simulink model "missile71"  (Simulink 6.3)
settings: Solver=ode4  StartTime=0.0  StopTime=10.0  FixedStep=0.0001  RelTol=1e-3
values from neighbouring files (symbols this model uses):
  K2 = lfr(D11,D12,D21,D22,blk)    [ex_2_1.m]
  Ma = 2 + jj*(2/5)    [ex_6_5_loop.m]
undefined symbols (not defined in the file or in its folder): K1, K3, m0, m1, m2, m3, z0, z1, z2, z3
settings Model: Creator=magni  LastModifiedBy=magni  ExtModeTrigMode=oneshot  ExtModeArmWhenConnect=off  ExtModeAutoUpdateStatusClock=off  StrictBusMsg=None
settings DataIOCC: LimitDataPoints=off
settings OptimizationCC: BlockReduction=off  BooleanDataType=off
settings DebuggingCC: SolverPrmCheckMsg=none
settings HardwareCC: TargetUnknown=on

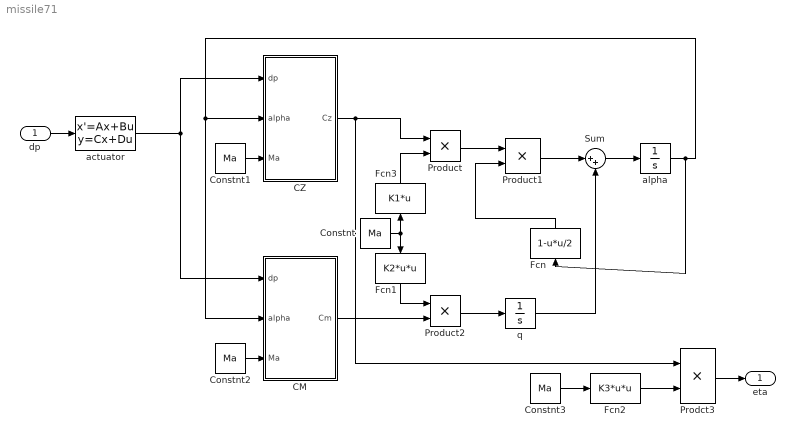
== system missile71 ==
  dp : Inport
  CM : Subsystem
  CZ : Subsystem
  Constnt{,1..3} (4 alike) : Constant  Value=Ma
  Fcn : Fcn  Orientation=up  Expr=1-u*u/2
  Fcn1 : Fcn  Orientation=down  Expr=K2*u*u
  Fcn2 : Fcn  Expr=K3*u*u
  Fcn3 : Fcn  Orientation=up  Expr=K1*u
  Prodct3 : Product  SaturateOnIntegerOverflow=on  RndMeth=Zero  InputSameDT=on
  Product : Product  SaturateOnIntegerOverflow=on  RndMeth=Zero  InputSameDT=on
  Product1 : Product  SaturateOnIntegerOverflow=on  RndMeth=Zero  InputSameDT=on
  Product2 : Product  SaturateOnIntegerOverflow=on  RndMeth=Zero  InputSameDT=on
  Sum : Sum  Inputs=|++  SaturateOnIntegerOverflow=on  InputSameDT=on
  actuator : StateSpace  A=[-210 -175.8;128 0]  B=[16;0]  C=[0 10.98]  D=0  X0=[0;0]
  alpha : Integrator
  q : Integrator
  eta : Outport
  wires:
  q/1 -> Sum/2
  Fcn3/1 -> Product/2
  Fcn/1 -> Product1/2
  Product/1 -> Product1/1
  Product1/1 -> Sum/1
  Sum/1 -> alpha/1
  Fcn1/1 -> Product2/1
  CM/1(Cm) -> Product2/2
  Product2/1 -> q/1
  CZ/1(Cz) -> Product/1, Prodct3/1
  alpha/1 -> CM/2(alpha), CZ/2(alpha), Fcn/1
  Fcn2/1 -> Prodct3/2
  Constnt3/1 -> Fcn2/1
  Constnt1/1 -> CZ/3(Ma)
  Constnt/1 -> Fcn3/1, Fcn1/1
  Constnt2/1 -> CM/3(Ma)
  Prodct3/1 -> eta/1
  dp/1 -> actuator/1
  actuator/1 -> CM/1(dp), CZ/1(dp)

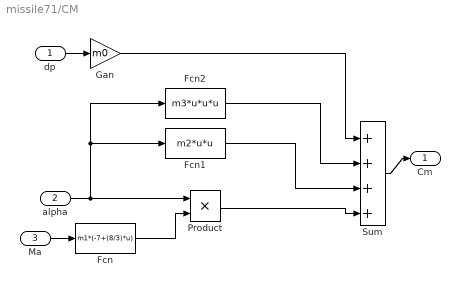
== system missile71/CM ==
  dp : Inport
  alpha : Inport  Port=2
  Ma : Inport  Port=3
  Fcn : Fcn  Expr=m1*(-7+(8/3)*u)
  Fcn1 : Fcn  Expr=m2*u*u
  Fcn2 : Fcn  Expr=m3*u*u*u
  Gan : Gain  Gain=m0  SaturateOnIntegerOverflow=on
  Product : Product  SaturateOnIntegerOverflow=on  RndMeth=Zero  InputSameDT=on
  Sum : Sum  Inputs=|++++  SaturateOnIntegerOverflow=on  InputSameDT=on
  Cm : Outport
  wires:
  Ma/1 -> Fcn/1
  Sum/1 -> Cm/1
  dp/1 -> Gan/1
  Product/1 -> Sum/4
  Fcn1/1 -> Sum/3
  Fcn2/1 -> Sum/2
  Gan/1 -> Sum/1
  alpha/1 -> Fcn2/1, Fcn1/1, Product/1
  Fcn/1 -> Product/2

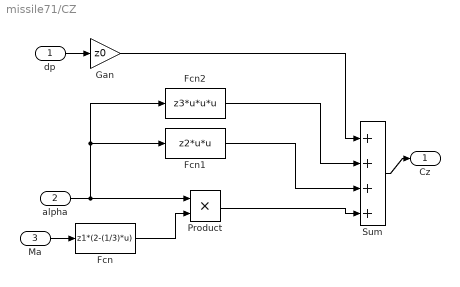
== system missile71/CZ ==
  dp : Inport
  alpha : Inport  Port=2
  Ma : Inport  Port=3
  Fcn : Fcn  Expr=z1*(2-(1/3)*u)
  Fcn1 : Fcn  Expr=z2*u*u
  Fcn2 : Fcn  Expr=z3*u*u*u
  Gan : Gain  Gain=z0  SaturateOnIntegerOverflow=on
  Product : Product  SaturateOnIntegerOverflow=on  RndMeth=Zero  InputSameDT=on
  Sum : Sum  Inputs=|++++  SaturateOnIntegerOverflow=on  InputSameDT=on
  Cz : Outport
  wires:
  Ma/1 -> Fcn/1
  Sum/1 -> Cz/1
  dp/1 -> Gan/1
  Product/1 -> Sum/4
  Fcn1/1 -> Sum/3
  Fcn2/1 -> Sum/2
  Gan/1 -> Sum/1
  alpha/1 -> Fcn2/1, Fcn1/1, Product/1
  Fcn/1 -> Product/2
